simulink model "MultipleAgentsChoice_NoVR"  (Simulink 7.5)
settings: Solver=ode45  StartTime=0.0  StopTime=1000  RelTol=1e-4  AbsTol=1e-4
libraries: simulink x64
(part 6 of 6)

== system MultipleAgentsChoice_NoVR/StatePropagation/SatelliteControlAccel/Agent Body2/Actual Thruster response/Xthruster/Thruster1/ThrustBlock/Voltage/Current ==
  Short? : Inport  OutDataType=sfix(16)  OutScaling=2^0
  MainSwitch : Inport  Port=2  OutDataType=sfix(16)  OutScaling=2^0
  Feed? : Inport  Port=3  OutDataType=sfix(16)  OutScaling=2^0
  Demux : Demux  Outputs=2
  MATLAB Fcn : MATLABFcn  MATLABFcn=ThrusterData  OutputDimensions=2
  Mux : Mux  Inputs=3
  Voltage : Outport  OutDataType=sfix(16)  OutScaling=2^0
  Current : Outport  Port=2  OutDataType=sfix(16)  OutScaling=2^0
  wires:
  Short?/1 -> Mux/1
  MainSwitch/1 -> Mux/2
  Feed?/1 -> Mux/3
  Mux/1 -> MATLAB Fcn/1
  MATLAB Fcn/1 -> Demux/1
  Demux/1 -> Voltage/1
  Demux/2 -> Current/1

== system MultipleAgentsChoice_NoVR/StatePropagation/SatelliteControlAccel/Agent Body2/Actual Thruster response/Ythruster1/Thruster1/ForceShort/S/C Conditioning ==
  SC : Inport  OutDataType=sfix(16)  OutScaling=2^0
  MainSwitch : Inport  Port=2  OutDataType=sfix(16)  OutScaling=2^0
  Constant : Constant  Value=2  OutDataType=sfix(16)  OutScaling=2^0
  Data Type Conversion : DataTypeConversion  OutDataType=sfix(16)  OutScaling=2^0
  Detect Decrease : simulink/Logic and Bit Operations/Detect Decrease  SystemSampleTime=-1  vinit=0
  Multiport Switch : MultiPortSwitch  DataPortOrder=Zero-based contiguous  Inputs=2  zeroidx=on
  Short? : Outport  OutDataType=sfix(16)  OutScaling=2^0
  wires:
  Multiport Switch/1 -> Short?/1
  Constant/1 -> Multiport Switch/3
  SC/1 -> Multiport Switch/2
  Data Type Conversion/1 -> Multiport Switch/1
  Detect Decrease/1 -> Data Type Conversion/1
  MainSwitch/1 -> Detect Decrease/1

== system MultipleAgentsChoice_NoVR/StatePropagation/SatelliteControlAccel/Agent Body2/Actual Thruster response/Ythruster1/Thruster1/ThrustBlock/ActiveThruster (logical) ==
  Short? : Inport  OutDataType=sfix(16)  OutScaling=2^0
  ThrusterOn? : Inport  Port=2  OutDataType=sfix(16)  OutScaling=2^0
  Feed? : Inport  Port=3  OutDataType=sfix(16)  OutScaling=2^0
  MATLAB Fcn : MATLABFcn  MATLABFcn=ActiveThruster  OutputDimensions=1
  Mux : Mux  Inputs=3
  Active : Outport  OutDataType=sfix(16)  OutScaling=2^0
  wires:
  MATLAB Fcn/1 -> Active/1
  Mux/1 -> MATLAB Fcn/1
  Feed?/1 -> Mux/3
  ThrusterOn?/1 -> Mux/2
  Short?/1 -> Mux/1

== system MultipleAgentsChoice_NoVR/StatePropagation/SatelliteControlAccel/Agent Body2/Actual Thruster response/Ythruster1/Thruster1/ThrustBlock/Voltage/Current ==
  Short? : Inport  OutDataType=sfix(16)  OutScaling=2^0
  MainSwitch : Inport  Port=2  OutDataType=sfix(16)  OutScaling=2^0
  Feed? : Inport  Port=3  OutDataType=sfix(16)  OutScaling=2^0
  Demux : Demux  Outputs=2
  MATLAB Fcn : MATLABFcn  MATLABFcn=ThrusterData  OutputDimensions=2
  Mux : Mux  Inputs=3
  Voltage : Outport  OutDataType=sfix(16)  OutScaling=2^0
  Current : Outport  Port=2  OutDataType=sfix(16)  OutScaling=2^0
  wires:
  Demux/2 -> Current/1
  Demux/1 -> Voltage/1
  MATLAB Fcn/1 -> Demux/1
  Mux/1 -> MATLAB Fcn/1
  Feed?/1 -> Mux/3
  MainSwitch/1 -> Mux/2
  Short?/1 -> Mux/1

== system MultipleAgentsChoice_NoVR/StatePropagation/SatelliteControlAccel/Agent Body2/Actual Thruster response/Zthruster1/Thruster1/ForceShort/S/C Conditioning ==
  SC : Inport  OutDataType=sfix(16)  OutScaling=2^0
  MainSwitch : Inport  Port=2  OutDataType=sfix(16)  OutScaling=2^0
  Constant : Constant  Value=2  OutDataType=sfix(16)  OutScaling=2^0
  Data Type Conversion : DataTypeConversion  OutDataType=sfix(16)  OutScaling=2^0
  Detect Decrease : simulink/Logic and Bit Operations/Detect Decrease  SystemSampleTime=-1  vinit=0
  Multiport Switch : MultiPortSwitch  DataPortOrder=Zero-based contiguous  Inputs=2  zeroidx=on
  Short? : Outport  OutDataType=sfix(16)  OutScaling=2^0
  wires:
  MainSwitch/1 -> Detect Decrease/1
  Detect Decrease/1 -> Data Type Conversion/1
  Data Type Conversion/1 -> Multiport Switch/1
  SC/1 -> Multiport Switch/2
  Constant/1 -> Multiport Switch/3
  Multiport Switch/1 -> Short?/1

== system MultipleAgentsChoice_NoVR/StatePropagation/SatelliteControlAccel/Agent Body2/Actual Thruster response/Zthruster1/Thruster1/ThrustBlock/ActiveThruster (logical) ==
  Short? : Inport  OutDataType=sfix(16)  OutScaling=2^0
  ThrusterOn? : Inport  Port=2  OutDataType=sfix(16)  OutScaling=2^0
  Feed? : Inport  Port=3  OutDataType=sfix(16)  OutScaling=2^0
  MATLAB Fcn : MATLABFcn  MATLABFcn=ActiveThruster  OutputDimensions=1
  Mux : Mux  Inputs=3
  Active : Outport  OutDataType=sfix(16)  OutScaling=2^0
  wires:
  Short?/1 -> Mux/1
  ThrusterOn?/1 -> Mux/2
  Feed?/1 -> Mux/3
  Mux/1 -> MATLAB Fcn/1
  MATLAB Fcn/1 -> Active/1

== system MultipleAgentsChoice_NoVR/StatePropagation/SatelliteControlAccel/Agent Body2/Actual Thruster response/Zthruster1/Thruster1/ThrustBlock/Voltage/Current ==
  Short? : Inport  OutDataType=sfix(16)  OutScaling=2^0
  MainSwitch : Inport  Port=2  OutDataType=sfix(16)  OutScaling=2^0
  Feed? : Inport  Port=3  OutDataType=sfix(16)  OutScaling=2^0
  Demux : Demux  Outputs=2
  MATLAB Fcn : MATLABFcn  MATLABFcn=ThrusterData  OutputDimensions=2
  Mux : Mux  Inputs=3
  Voltage : Outport  OutDataType=sfix(16)  OutScaling=2^0
  Current : Outport  Port=2  OutDataType=sfix(16)  OutScaling=2^0
  wires:
  Short?/1 -> Mux/1
  MainSwitch/1 -> Mux/2
  Feed?/1 -> Mux/3
  Mux/1 -> MATLAB Fcn/1
  MATLAB Fcn/1 -> Demux/1
  Demux/1 -> Voltage/1
  Demux/2 -> Current/1

== system MultipleAgentsChoice_NoVR/StatePropagation/SatelliteControlAccel/Agent Body3/Actual Thruster response/XYZthruster/Thruster1/ForceShort/S/C Conditioning ==
  SC : Inport  OutDataType=sfix(16)  OutScaling=2^0
  MainSwitch : Inport  Port=2  OutDataType=sfix(16)  OutScaling=2^0
  Constant : Constant  Value=2  OutDataType=sfix(16)  OutScaling=2^0
  Data Type Conversion : DataTypeConversion  OutDataType=sfix(16)  OutScaling=2^0
  Detect Decrease : simulink/Logic and Bit Operations/Detect Decrease  SystemSampleTime=-1  vinit=0
  Multiport Switch : MultiPortSwitch  DataPortOrder=Zero-based contiguous  Inputs=2  zeroidx=on
  Short? : Outport  OutDataType=sfix(16)  OutScaling=2^0
  wires:
  Multiport Switch/1 -> Short?/1
  Constant/1 -> Multiport Switch/3
  SC/1 -> Multiport Switch/2
  Data Type Conversion/1 -> Multiport Switch/1
  Detect Decrease/1 -> Data Type Conversion/1
  MainSwitch/1 -> Detect Decrease/1

== system MultipleAgentsChoice_NoVR/StatePropagation/SatelliteControlAccel/Agent Body3/Actual Thruster response/XYZthruster/Thruster1/ThrustBlock/ActiveThruster (logical) ==
  Short? : Inport  OutDataType=sfix(16)  OutScaling=2^0
  ThrusterOn? : Inport  Port=2  OutDataType=sfix(16)  OutScaling=2^0
  Feed? : Inport  Port=3  OutDataType=sfix(16)  OutScaling=2^0
  MATLAB Fcn : MATLABFcn  MATLABFcn=ActiveThruster  OutputDimensions=1
  Mux : Mux  Inputs=3
  Active : Outport  OutDataType=sfix(16)  OutScaling=2^0
  wires:
  MATLAB Fcn/1 -> Active/1
  Mux/1 -> MATLAB Fcn/1
  Feed?/1 -> Mux/3
  ThrusterOn?/1 -> Mux/2
  Short?/1 -> Mux/1

== system MultipleAgentsChoice_NoVR/StatePropagation/SatelliteControlAccel/Agent Body3/Actual Thruster response/XYZthruster/Thruster1/ThrustBlock/Voltage/Current ==
  Short? : Inport  OutDataType=sfix(16)  OutScaling=2^0
  MainSwitch : Inport  Port=2  OutDataType=sfix(16)  OutScaling=2^0
  Feed? : Inport  Port=3  OutDataType=sfix(16)  OutScaling=2^0
  Demux : Demux  Outputs=2
  MATLAB Fcn : MATLABFcn  MATLABFcn=ThrusterData  OutputDimensions=2
  Mux : Mux  Inputs=3
  Voltage : Outport  OutDataType=sfix(16)  OutScaling=2^0
  Current : Outport  Port=2  OutDataType=sfix(16)  OutScaling=2^0
  wires:
  Demux/2 -> Current/1
  Demux/1 -> Voltage/1
  MATLAB Fcn/1 -> Demux/1
  Mux/1 -> MATLAB Fcn/1
  Feed?/1 -> Mux/3
  MainSwitch/1 -> Mux/2
  Short?/1 -> Mux/1

== system MultipleAgentsChoice_NoVR/StatePropagation/SatelliteControlAccel/Agent Body3/Actual Thruster response/Xthruster/Thruster1/ForceShort/S/C Conditioning ==
  SC : Inport  OutDataType=sfix(16)  OutScaling=2^0
  MainSwitch : Inport  Port=2  OutDataType=sfix(16)  OutScaling=2^0
  Constant : Constant  Value=2  OutDataType=sfix(16)  OutScaling=2^0
  Data Type Conversion : DataTypeConversion  OutDataType=sfix(16)  OutScaling=2^0
  Detect Decrease : simulink/Logic and Bit Operations/Detect Decrease  SystemSampleTime=-1  vinit=0
  Multiport Switch : MultiPortSwitch  DataPortOrder=Zero-based contiguous  Inputs=2  zeroidx=on
  Short? : Outport  OutDataType=sfix(16)  OutScaling=2^0
  wires:
  MainSwitch/1 -> Detect Decrease/1
  Detect Decrease/1 -> Data Type Conversion/1
  Data Type Conversion/1 -> Multiport Switch/1
  SC/1 -> Multiport Switch/2
  Constant/1 -> Multiport Switch/3
  Multiport Switch/1 -> Short?/1

== system MultipleAgentsChoice_NoVR/StatePropagation/SatelliteControlAccel/Agent Body3/Actual Thruster response/Xthruster/Thruster1/ThrustBlock/ActiveThruster (logical) ==
  Short? : Inport  OutDataType=sfix(16)  OutScaling=2^0
  ThrusterOn? : Inport  Port=2  OutDataType=sfix(16)  OutScaling=2^0
  Feed? : Inport  Port=3  OutDataType=sfix(16)  OutScaling=2^0
  MATLAB Fcn : MATLABFcn  MATLABFcn=ActiveThruster  OutputDimensions=1
  Mux : Mux  Inputs=3
  Active : Outport  OutDataType=sfix(16)  OutScaling=2^0
  wires:
  Short?/1 -> Mux/1
  ThrusterOn?/1 -> Mux/2
  Feed?/1 -> Mux/3
  Mux/1 -> MATLAB Fcn/1
  MATLAB Fcn/1 -> Active/1

== system MultipleAgentsChoice_NoVR/StatePropagation/SatelliteControlAccel/Agent Body3/Actual Thruster response/Xthruster/Thruster1/ThrustBlock/Voltage/Current ==
  Short? : Inport  OutDataType=sfix(16)  OutScaling=2^0
  MainSwitch : Inport  Port=2  OutDataType=sfix(16)  OutScaling=2^0
  Feed? : Inport  Port=3  OutDataType=sfix(16)  OutScaling=2^0
  Demux : Demux  Outputs=2
  MATLAB Fcn : MATLABFcn  MATLABFcn=ThrusterData  OutputDimensions=2
  Mux : Mux  Inputs=3
  Voltage : Outport  OutDataType=sfix(16)  OutScaling=2^0
  Current : Outport  Port=2  OutDataType=sfix(16)  OutScaling=2^0
  wires:
  Short?/1 -> Mux/1
  MainSwitch/1 -> Mux/2
  Feed?/1 -> Mux/3
  Mux/1 -> MATLAB Fcn/1
  MATLAB Fcn/1 -> Demux/1
  Demux/1 -> Voltage/1
  Demux/2 -> Current/1

== system MultipleAgentsChoice_NoVR/StatePropagation/SatelliteControlAccel/Agent Body3/Actual Thruster response/Ythruster1/Thruster1/ForceShort/S/C Conditioning ==
  SC : Inport  OutDataType=sfix(16)  OutScaling=2^0
  MainSwitch : Inport  Port=2  OutDataType=sfix(16)  OutScaling=2^0
  Constant : Constant  Value=2  OutDataType=sfix(16)  OutScaling=2^0
  Data Type Conversion : DataTypeConversion  OutDataType=sfix(16)  OutScaling=2^0
  Detect Decrease : simulink/Logic and Bit Operations/Detect Decrease  SystemSampleTime=-1  vinit=0
  Multiport Switch : MultiPortSwitch  DataPortOrder=Zero-based contiguous  Inputs=2  zeroidx=on
  Short? : Outport  OutDataType=sfix(16)  OutScaling=2^0
  wires:
  Multiport Switch/1 -> Short?/1
  Constant/1 -> Multiport Switch/3
  SC/1 -> Multiport Switch/2
  Data Type Conversion/1 -> Multiport Switch/1
  Detect Decrease/1 -> Data Type Conversion/1
  MainSwitch/1 -> Detect Decrease/1

== system MultipleAgentsChoice_NoVR/StatePropagation/SatelliteControlAccel/Agent Body3/Actual Thruster response/Ythruster1/Thruster1/ThrustBlock/ActiveThruster (logical) ==
  Short? : Inport  OutDataType=sfix(16)  OutScaling=2^0
  ThrusterOn? : Inport  Port=2  OutDataType=sfix(16)  OutScaling=2^0
  Feed? : Inport  Port=3  OutDataType=sfix(16)  OutScaling=2^0
  MATLAB Fcn : MATLABFcn  MATLABFcn=ActiveThruster  OutputDimensions=1
  Mux : Mux  Inputs=3
  Active : Outport  OutDataType=sfix(16)  OutScaling=2^0
  wires:
  MATLAB Fcn/1 -> Active/1
  Mux/1 -> MATLAB Fcn/1
  Feed?/1 -> Mux/3
  ThrusterOn?/1 -> Mux/2
  Short?/1 -> Mux/1

== system MultipleAgentsChoice_NoVR/StatePropagation/SatelliteControlAccel/Agent Body3/Actual Thruster response/Ythruster1/Thruster1/ThrustBlock/Voltage/Current ==
  Short? : Inport  OutDataType=sfix(16)  OutScaling=2^0
  MainSwitch : Inport  Port=2  OutDataType=sfix(16)  OutScaling=2^0
  Feed? : Inport  Port=3  OutDataType=sfix(16)  OutScaling=2^0
  Demux : Demux  Outputs=2
  MATLAB Fcn : MATLABFcn  MATLABFcn=ThrusterData  OutputDimensions=2
  Mux : Mux  Inputs=3
  Voltage : Outport  OutDataType=sfix(16)  OutScaling=2^0
  Current : Outport  Port=2  OutDataType=sfix(16)  OutScaling=2^0
  wires:
  Demux/2 -> Current/1
  Demux/1 -> Voltage/1
  MATLAB Fcn/1 -> Demux/1
  Mux/1 -> MATLAB Fcn/1
  Feed?/1 -> Mux/3
  MainSwitch/1 -> Mux/2
  Short?/1 -> Mux/1

== system MultipleAgentsChoice_NoVR/StatePropagation/SatelliteControlAccel/Agent Body3/Actual Thruster response/Zthruster1/Thruster1/ForceShort/S/C Conditioning ==
  SC : Inport  OutDataType=sfix(16)  OutScaling=2^0
  MainSwitch : Inport  Port=2  OutDataType=sfix(16)  OutScaling=2^0
  Constant : Constant  Value=2  OutDataType=sfix(16)  OutScaling=2^0
  Data Type Conversion : DataTypeConversion  OutDataType=sfix(16)  OutScaling=2^0
  Detect Decrease : simulink/Logic and Bit Operations/Detect Decrease  SystemSampleTime=-1  vinit=0
  Multiport Switch : MultiPortSwitch  DataPortOrder=Zero-based contiguous  Inputs=2  zeroidx=on
  Short? : Outport  OutDataType=sfix(16)  OutScaling=2^0
  wires:
  MainSwitch/1 -> Detect Decrease/1
  Detect Decrease/1 -> Data Type Conversion/1
  Data Type Conversion/1 -> Multiport Switch/1
  SC/1 -> Multiport Switch/2
  Constant/1 -> Multiport Switch/3
  Multiport Switch/1 -> Short?/1

== system MultipleAgentsChoice_NoVR/StatePropagation/SatelliteControlAccel/Agent Body3/Actual Thruster response/Zthruster1/Thruster1/ThrustBlock/ActiveThruster (logical) ==
  Short? : Inport  OutDataType=sfix(16)  OutScaling=2^0
  ThrusterOn? : Inport  Port=2  OutDataType=sfix(16)  OutScaling=2^0
  Feed? : Inport  Port=3  OutDataType=sfix(16)  OutScaling=2^0
  MATLAB Fcn : MATLABFcn  MATLABFcn=ActiveThruster  OutputDimensions=1
  Mux : Mux  Inputs=3
  Active : Outport  OutDataType=sfix(16)  OutScaling=2^0
  wires:
  Short?/1 -> Mux/1
  ThrusterOn?/1 -> Mux/2
  Feed?/1 -> Mux/3
  Mux/1 -> MATLAB Fcn/1
  MATLAB Fcn/1 -> Active/1

== system MultipleAgentsChoice_NoVR/StatePropagation/SatelliteControlAccel/Agent Body3/Actual Thruster response/Zthruster1/Thruster1/ThrustBlock/Voltage/Current ==
  Short? : Inport  OutDataType=sfix(16)  OutScaling=2^0
  MainSwitch : Inport  Port=2  OutDataType=sfix(16)  OutScaling=2^0
  Feed? : Inport  Port=3  OutDataType=sfix(16)  OutScaling=2^0
  Demux : Demux  Outputs=2
  MATLAB Fcn : MATLABFcn  MATLABFcn=ThrusterData  OutputDimensions=2
  Mux : Mux  Inputs=3
  Voltage : Outport  OutDataType=sfix(16)  OutScaling=2^0
  Current : Outport  Port=2  OutDataType=sfix(16)  OutScaling=2^0
  wires:
  Short?/1 -> Mux/1
  MainSwitch/1 -> Mux/2
  Feed?/1 -> Mux/3
  Mux/1 -> MATLAB Fcn/1
  MATLAB Fcn/1 -> Demux/1
  Demux/1 -> Voltage/1
  Demux/2 -> Current/1
